simulink model "fifo"  (R2015a)
settings: Solver=ode45  StartTime=0.0  StopTime=10.0  RelTol=1e-3
InitFcn:
  | %% DSPBuilder Start
  | alt_dspbuilder_update_model(bdroot)
  | %% DSPBuilder End
libraries: allblocks_alteradspbuilder2 x5
settings Model: Creator=ASUS  LastModifiedBy=ASUS

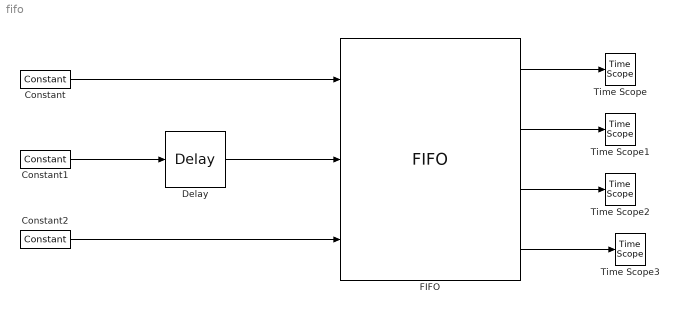
== system fifo ==
  Constant : allblocks_alteradspbuilder2/Constant  mask_cst=5  BusType=Unsigned Integer  bwl=8  bwr=0  roundMode=Truncate  satMode=Wrap  SpecifyClock=off  allowFloatingPointOverride=on  logOutputs=off  logFile=C:\Users\ASUS\Desktop\final_sift_fpga\tb_fifo\fifo_Constant.fixedpointlog
  Constant1 : allblocks_alteradspbuilder2/Constant  mask_cst=1  BusType=Single Bit  bwl=8  bwr=0  roundMode=Truncate  satMode=Wrap  SpecifyClock=off  allowFloatingPointOverride=on  logOutputs=off  logFile=C:\Users\ASUS\Desktop\final_sift_fpga\tb_fifo\fifo_Constant1.fixedpointlog
  Constant2 : allblocks_alteradspbuilder2/Constant  mask_cst=1  BusType=Single Bit  bwl=8  bwr=0  roundMode=Truncate  satMode=Wrap  SpecifyClock=off  allowFloatingPointOverride=on  logOutputs=off  logFile=C:\Users\ASUS\Desktop\final_sift_fpga\tb_fifo\fifo_Constant2.fixedpointlog
  Delay : allblocks_alteradspbuilder2/Delay  pipeline=5  pipeline_display=5  ClockPhase=1  use_ena=off  use_sclr=off  allowFloatingPointOverride=on  logOutputs=off  logFile=C:\Users\ASUS\Desktop\final_sift_fpga\tb_fifo\fifo_Delay.fixedpointlog  use_init=off  reset_value=1
  FIFO : allblocks_alteradspbuilder2/FIFO  numwords=64  BusType=Unsigned Integer  bwl=8  bwr=0  ram_type=AUTO  use_sclr=off  use_les_only=off  showahead_mode=off  allowFloatingPointOverride=on  logOutputs=off  logFile=C:\Users\ASUS\Desktop\final_sift_fpga\tb_fifo\fifo_FIFO%3A%3Aq.fixedpointlog,C:\Users\ASUS\Desktop\final_sift_fpga\tb_fifo\fifo_FIFO%3A%3Afull.fixedpointlog,C:\Users\ASUS\Desktop\final_sift_fpga\tb_fifo\fifo_FIFO%3A%3Aempty.fixedpointlog,C:\Users\ASUS\Desktop\final_sift_fpga\tb_fifo\fifo_FIFO%3A%3Ausedw.fixedpointlog,
  Time Scope{,1..3} (4 alike) : TimeScope  DefaultConfigurationName=spbscopes.TimeScopeBlockCfg
  wires:
  Constant/1 -> FIFO/1
  Constant1/1 -> Delay/1
  FIFO/2 -> Time Scope1/1
  FIFO/1 -> Time Scope/1
  FIFO/3 -> Time Scope2/1
  FIFO/4 -> Time Scope3/1
  Constant2/1 -> FIFO/3
  Delay/1 -> FIFO/2
